simulink model "sf_multfuncout"  (Simulink 6.0)
settings: Solver=ode45  StartTime=0.0  StopTime=30  MaxStep=1  RelTol=1e-3
settings Model: CovMetricSettings=dcmtr  Creator=The MathWorks Inc.  LastModifiedBy=batserve  ExtModeAutoUpdateStatusClock=off
settings OptimizationCC: BooleanDataType=off
settings DebuggingCC: CheckExecutionContextPreStartOutputMsg=on  CheckExecutionContextRuntimeOutputMsg=on  SolverPrmCheckMsg=none
settings HardwareCC: TargetUnknown=on

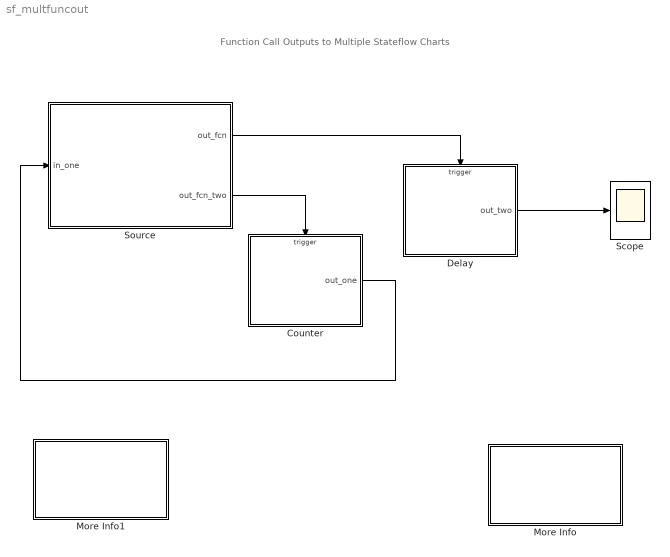
== system sf_multfuncout ==
  note: Function Call Outputs to Multiple Stateflow Charts
  Counter : Stateflow chart  TreatAsAtomicUnit=on  PropExecContextAcrossSSBoundary=on
  Delay : Stateflow chart  TreatAsAtomicUnit=on  PropExecContextAcrossSSBoundary=on
  More Info : Subsystem  PropExecContextAcrossSSBoundary=on
      mask Display: disp('Double click\nhere for\ninformation on\nthis demonstration')
  More Info1 : Subsystem  PropExecContextAcrossSSBoundary=on
      settings: OpenFcn=simcad(bdroot);
      mask Display: disp('Double click\nhere for\nSimulink\Stateflow\n Help')
  Scope : Scope
      settings: TimeRange=30  YMin=0  YMax=7
  Source : Stateflow chart  PropExecContextAcrossSSBoundary=on
  wires:
  Source/2(out_fcn_two) -> Counter/Trigger
  Source/1(out_fcn) -> Delay/Trigger
  Delay/1(out_two) -> Scope/1
  Counter/1(out_one) -> Source/1(in_one)

== system sf_multfuncout/More Info ==
  note: The main purpose of this demonstration is to illustrate the use of feedback when using function-call
      | outputs. The 'Source' chart sends the signal 'out_fcn_two' when transition to from State A to State B or
      | vice versa. 'out_fcn_two' activates 'Counter' everytime it is sent out. 'Counter' also sends out a data
      | output, 'out_one' which is fed back to 'Source' as data 'Input from Simulink'. If the source is in State B,
      | then a transition is taken from State B to State C if 'out_one' is greater than 10. If this transition is taken,
      | then a new function-call event, 'out_fcn' is sent to the 'Delay' chart. The 'Delay' chart simply adds a 1
      | to its output, 'out_two' everytime it is activated. In the output, 'Scope', notice that there is an initial delay
      | that is the time it takes for the first 'out_fcn' to be sent.
  note: Function Call Outputs

== system sf_multfuncout/More Info1 ==

== stateflow chart Source ==
  state A
  state B
  state C
  A -> B : /out_fcn_two;
  B -> A : /out_fcn_two;
  (default) -> A
  B -> C : [in_one>10]/out_fcn;
  C -> A
  data: local_count local double; in_one input double
  events: out_fcn output FUNCTION_CALL_EVENT; out_fcn_two output FUNCTION_CALL_EVENT

== stateflow chart Counter ==
  state A
    en:out_one=1;
    du:out_one++;
  (default) -> A
  data: out_one output double
  events: event input FUNCTION_CALL_EVENT

== stateflow chart Delay ==
  state A
    en:out_two=1;
    du:out_two++;
  (default) -> A
  data: out_two output double
  events: event input FUNCTION_CALL_EVENT
